simulink library "halin"  (R2021b)
settings: Solver=VariableStepAuto  StartTime=0.0  StopTime=10.0  RelTol=1e-3
undefined symbols (not defined in the file): KHAL_CAN1ABM1E2E_flg, KHAL_CAN1ESC1E2E_flg, KHAL_CAN1ESC5E2E_flg, KHAL_CAN1ESC7E2E_flg, KHAL_CAN1FCM2E2E_flg, KHAL_CAN1FCM3E2E_flg, KHAL_CAN1FCM4E2E_flg, KHAL_CAN3BMS1E2E_flg, KHAL_CAN3BMS6E2E_flg, KHAL_CAN3CCU1E2E_flg, KHAL_CAN3CCU2E2E_flg, KHAL_CAN3MCUF1E2E_flg, KHAL_CAN3MCUR1E2E_flg, KHAL_CAN3Shifter1E2E_flg, TRUE
libraries: simulink x420, FVT_lib x149, hcu_lib x49
(part 3 of 14)

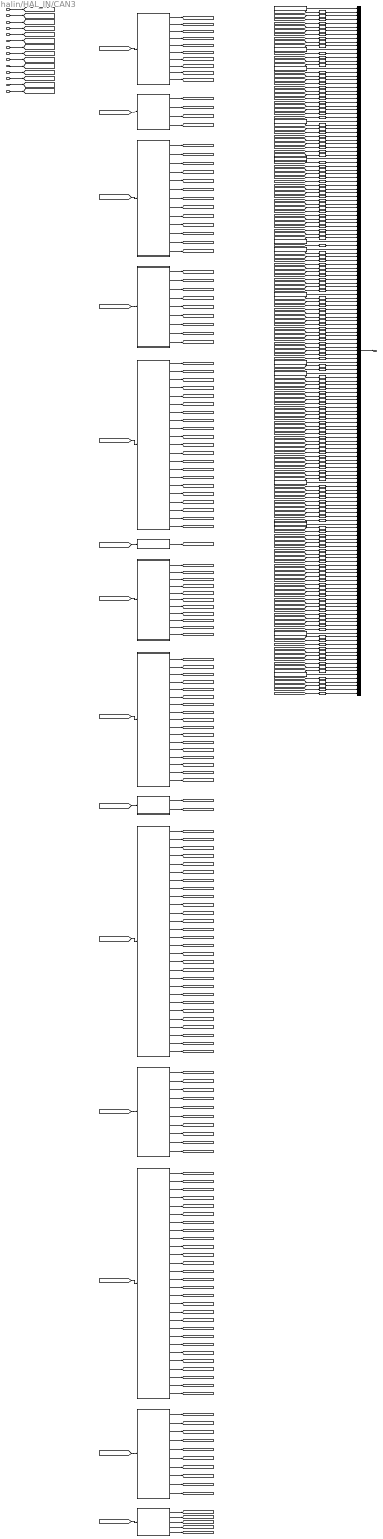
== system halin/HAL_IN/CAN3 ==
  DT_CAN3_SG_BMS1 : Inport
  DT_CAN3_SG_BMS2 : Inport  Port=2
  DT_CAN3_SG_BMS3 : Inport  Port=3
  DT_CAN3_SG_BMS4 : Inport  Port=4
  DT_CAN3_SG_BMS6 : Inport  Port=5
  DT_CAN3_SG_BMS7 : Inport  Port=6
  DT_CAN3_SG_CCU1 : Inport  Port=7
  DT_CAN3_SG_CCU2 : Inport  Port=8
  DT_CAN3_SG_CCU4 : Inport  Port=9
  DT_CAN3_SG_MCU_F1 : Inport  Port=10
  DT_CAN3_SG_MCU_F2 : Inport  Port=11
  DT_CAN3_SG_MCU_R1 : Inport  Port=12
  DT_CAN3_SG_MCU_R2 : Inport  Port=13
  DT_CAN3_SG_Shifter1 : Inport  Port=14
  BMS1 : Subsystem
  BMS2 : Subsystem
  BMS3 : Subsystem
  BMS4 : Subsystem
  BMS6 : Subsystem
  BMS7 : Subsystem
  CCU1 : Subsystem
  CCU2 : Subsystem
  CCU4 : Subsystem
  MCU_F1 : Subsystem
  MCU_F2 : Subsystem
  MCU_R1 : Subsystem
  MCU_R2 : Subsystem
  Shifter1 : Subsystem
  UnitConverter{,1,36..37,40..48,51..52,55,57..59,67,69..70,72,74,78,80..81,88..92,101..102,104..106,126..127,129..131,140..141,143..145,164..165} (49 alike) : DataTypeConversion  OutDataTypeStr=boolean
  UnitConverter{4..31,61..62,64..65,75..77,82,86..87,93,95,98..100,108..114,116..117,122..123,132,134,137..139,147..155,160..161} (70 alike) : DataTypeConversion  OutDataTypeStr=single
  UnitConverter{2..3,32..35,38..39,49..50,53..54,56,60,63,66,68,71,73,79,83..85,94,96..97,103,107,115,118..121,124..125,128,133,135..136,142,146,156..159,162..163,166..168} (50 alike) : DataTypeConversion  OutDataTypeStr=uint8
  VHAL_CANMsgInvalidBMS1_flg : Subsystem  AncestorBlock=FVT_lib/hal/MsgTimeoutJudge_CAN_AUTOSAR
      mask help: MeasumentTrigerEvent
      mask Display: fprintf('MsgTimeoutJudge_CAN\nAUTOSAR');
  VHAL_CANMsgInvalidBMS2_flg : Subsystem  AncestorBlock=FVT_lib/hal/MsgTimeoutJudge_CAN_AUTOSAR
      mask help: MeasumentTrigerEvent
      mask Display: fprintf('MsgTimeoutJudge_CAN\nAUTOSAR');
  VHAL_CANMsgInvalidBMS3_flg : Subsystem  AncestorBlock=FVT_lib/hal/MsgTimeoutJudge_CAN_AUTOSAR
      mask help: MeasumentTrigerEvent
      mask Display: fprintf('MsgTimeoutJudge_CAN\nAUTOSAR');
  VHAL_CANMsgInvalidBMS4_flg : Subsystem  AncestorBlock=FVT_lib/hal/MsgTimeoutJudge_CAN_AUTOSAR
      mask help: MeasumentTrigerEvent
      mask Display: fprintf('MsgTimeoutJudge_CAN\nAUTOSAR');
  VHAL_CANMsgInvalidBMS6_flg : Subsystem  AncestorBlock=FVT_lib/hal/MsgTimeoutJudge_CAN_AUTOSAR
      mask help: MeasumentTrigerEvent
      mask Display: fprintf('MsgTimeoutJudge_CAN\nAUTOSAR');
  VHAL_CANMsgInvalidBMS7_flg : Subsystem  AncestorBlock=FVT_lib/hal/MsgTimeoutJudge_CAN_AUTOSAR
      mask help: MeasumentTrigerEvent
      mask Display: fprintf('MsgTimeoutJudge_CAN\nAUTOSAR');
  VHAL_CANMsgInvalidCCU1_flg : Subsystem  AncestorBlock=FVT_lib/hal/MsgTimeoutJudge_CAN_AUTOSAR
      mask help: MeasumentTrigerEvent
      mask Display: fprintf('MsgTimeoutJudge_CAN\nAUTOSAR');
  VHAL_CANMsgInvalidCCU2_flg : Subsystem  AncestorBlock=FVT_lib/hal/MsgTimeoutJudge_CAN_AUTOSAR
      mask help: MeasumentTrigerEvent
      mask Display: fprintf('MsgTimeoutJudge_CAN\nAUTOSAR');
  VHAL_CANMsgInvalidCCU4_flg : Subsystem  AncestorBlock=FVT_lib/hal/MsgTimeoutJudge_CAN_AUTOSAR
      mask help: MeasumentTrigerEvent
      mask Display: fprintf('MsgTimeoutJudge_CAN\nAUTOSAR');
  VHAL_CANMsgInvalidMCUF1_flg : Subsystem  AncestorBlock=FVT_lib/hal/MsgTimeoutJudge_CAN_AUTOSAR
      mask help: MeasumentTrigerEvent
      mask Display: fprintf('MsgTimeoutJudge_CAN\nAUTOSAR');
  VHAL_CANMsgInvalidMCUF2_flg : Subsystem  AncestorBlock=FVT_lib/hal/MsgTimeoutJudge_CAN_AUTOSAR
      mask help: MeasumentTrigerEvent
      mask Display: fprintf('MsgTimeoutJudge_CAN\nAUTOSAR');
  VHAL_CANMsgInvalidMCUR1_flg : Subsystem  AncestorBlock=FVT_lib/hal/MsgTimeoutJudge_CAN_AUTOSAR
      mask help: MeasumentTrigerEvent
      mask Display: fprintf('MsgTimeoutJudge_CAN\nAUTOSAR');
  VHAL_CANMsgInvalidMCUR2_flg : Subsystem  AncestorBlock=FVT_lib/hal/MsgTimeoutJudge_CAN_AUTOSAR
      mask help: MeasumentTrigerEvent
      mask Display: fprintf('MsgTimeoutJudge_CAN\nAUTOSAR');
  VHAL_CANMsgInvalidShifter1_flg : Subsystem  AncestorBlock=FVT_lib/hal/MsgTimeoutJudge_CAN_AUTOSAR
      mask help: MeasumentTrigerEvent
      mask Display: fprintf('MsgTimeoutJudge_CAN\nAUTOSAR');
  bus_creator : BusCreator  Inputs=183
  HAL_CAN3_outputs : Outport
  wires:
  DT_CAN3_SG_BMS1/1 -> [DT_CAN3_SG_BMS1]
  DT_CAN3_SG_BMS2/1 -> [DT_CAN3_SG_BMS2]
  DT_CAN3_SG_BMS3/1 -> [DT_CAN3_SG_BMS3]
  DT_CAN3_SG_BMS4/1 -> [DT_CAN3_SG_BMS4]
  DT_CAN3_SG_BMS6/1 -> [DT_CAN3_SG_BMS6]
  DT_CAN3_SG_BMS7/1 -> [DT_CAN3_SG_BMS7]
  DT_CAN3_SG_CCU1/1 -> [DT_CAN3_SG_CCU1]
  DT_CAN3_SG_CCU2/1 -> [DT_CAN3_SG_CCU2]
  DT_CAN3_SG_CCU4/1 -> [DT_CAN3_SG_CCU4]
  DT_CAN3_SG_MCU_F1/1 -> [DT_CAN3_SG_MCU_F1]
  DT_CAN3_SG_MCU_F2/1 -> [DT_CAN3_SG_MCU_F2]
  DT_CAN3_SG_MCU_R1/1 -> [DT_CAN3_SG_MCU_R1]
  DT_CAN3_SG_MCU_R2/1 -> [DT_CAN3_SG_MCU_R2]
  DT_CAN3_SG_Shifter1/1 -> [DT_CAN3_SG_Shifter1]
  [DT_CAN3_SG_BMS1] -> BMS1/1(DT_CAN3_SG_BMS1)
  [DT_CAN3_SG_BMS2] -> BMS2/1(DT_CAN3_SG_BMS2)
  [DT_CAN3_SG_BMS3] -> BMS3/1(DT_CAN3_SG_BMS3)
  [DT_CAN3_SG_BMS4] -> BMS4/1(DT_CAN3_SG_BMS4)
  [DT_CAN3_SG_BMS6] -> BMS6/1(DT_CAN3_SG_BMS6)
  [DT_CAN3_SG_BMS7] -> BMS7/1(DT_CAN3_SG_BMS7)
  [DT_CAN3_SG_CCU1] -> CCU1/1(DT_CAN3_SG_CCU1)
  [DT_CAN3_SG_CCU2] -> CCU2/1(DT_CAN3_SG_CCU2)
  [DT_CAN3_SG_CCU4] -> CCU4/1(DT_CAN3_SG_CCU4)
  [DT_CAN3_SG_MCU_F1] -> MCU_F1/1(DT_CAN3_SG_MCU_F1)
  [DT_CAN3_SG_MCU_F2] -> MCU_F2/1(DT_CAN3_SG_MCU_F2)
  [DT_CAN3_SG_MCU_R1] -> MCU_R1/1(DT_CAN3_SG_MCU_R1)
  [DT_CAN3_SG_MCU_R2] -> MCU_R2/1(DT_CAN3_SG_MCU_R2)
  [DT_CAN3_SG_Shifter1] -> Shifter1/1(DT_CAN3_SG_Shifter1)
  bus_creator/1 -> HAL_CAN3_outputs/1
  VHAL_CANMsgInvalidBMS1_flg/1(Out) -> bus_creator/1
  BMS1/1(VHAL_BMS1CSErr_flg) -> [VHAL_BMS1CSErr_flg]
  UnitConverter/1 -> bus_creator/2  "VHAL_BMS1CSErr_flg"
  [VHAL_BMS1CSErr_flg] -> UnitConverter/1
  BMS1/2(VHAL_BMS1RCErr_flg) -> [VHAL_BMS1RCErr_flg]
  UnitConverter1/1 -> bus_creator/3  "VHAL_BMS1RCErr_flg"
  [VHAL_BMS1RCErr_flg] -> UnitConverter1/1
  BMS1/3(VHAL_BMSChckSum1_enum) -> [VHAL_BMSChckSum1_enum]
  UnitConverter2/1 -> bus_creator/4  "VHAL_BMSChckSum1_enum"
  [VHAL_BMSChckSum1_enum] -> UnitConverter2/1
  BMS1/4(VHAL_BMSRolCnct1_enum) -> [VHAL_BMSRolCnct1_enum]
  UnitConverter3/1 -> bus_creator/5  "VHAL_BMSRolCnct1_enum"
  [VHAL_BMSRolCnct1_enum] -> UnitConverter3/1
  BMS1/5(VHAL_HVBPwrAvailChrg_kW) -> [VHAL_HVBPwrAvailChrg_kW]
  UnitConverter4/1 -> bus_creator/6  "VHAL_HVBPwrAvailChrg_kW"
  [VHAL_HVBPwrAvailChrg_kW] -> UnitConverter4/1
  BMS1/6(VHAL_HVBPwrAvailChrg30_kW) -> [VHAL_HVBPwrAvailChrg30_kW]
  UnitConverter5/1 -> bus_creator/7  "VHAL_HVBPwrAvailChrg30_kW"
  [VHAL_HVBPwrAvailChrg30_kW] -> UnitConverter5/1
  BMS1/7(VHAL_HVBPwrAvailChrg60_kW) -> [VHAL_HVBPwrAvailChrg60_kW]
  UnitConverter6/1 -> bus_creator/8  "VHAL_HVBPwrAvailChrg60_kW"
  [VHAL_HVBPwrAvailChrg60_kW] -> UnitConverter6/1
  BMS1/8(VHAL_HVBPwrAvailDchrg_kW) -> [VHAL_HVBPwrAvailDchrg_kW]
  UnitConverter7/1 -> bus_creator/9  "VHAL_HVBPwrAvailDchrg_kW"
  [VHAL_HVBPwrAvailDchrg_kW] -> UnitConverter7/1
  BMS1/9(VHAL_HVBPwrAvailDchrg30_kW) -> [VHAL_HVBPwrAvailDchrg30_kW]
  UnitConverter8/1 -> bus_creator/10  "VHAL_HVBPwrAvailDchrg30_kW"
  [VHAL_HVBPwrAvailDchrg30_kW] -> UnitConverter8/1
  BMS1/10(VHAL_HVBPwrAvailDchrg60_kW) -> [VHAL_HVBPwrAvailDchrg60_kW]
  UnitConverter9/1 -> bus_creator/11  "VHAL_HVBPwrAvailDchrg60_kW"
  [VHAL_HVBPwrAvailDchrg60_kW] -> UnitConverter9/1
  VHAL_CANMsgInvalidBMS2_flg/1(Out) -> bus_creator/12
  BMS2/1(VHAL_HVInVolt_V) -> [VHAL_HVInVolt_V]
  UnitConverter10/1 -> bus_creator/13  "VHAL_HVInVolt_V"
  [VHAL_HVInVolt_V] -> UnitConverter10/1
  BMS2/2(VHAL_LVBattDet12V_V) -> [VHAL_LVBattDet12V_V]
  UnitConverter11/1 -> bus_creator/14  "VHAL_LVBattDet12V_V"
  [VHAL_LVBattDet12V_V] -> UnitConverter11/1
  BMS2/3(VHAL_OBCDCCurLm_A) -> [VHAL_OBCDCCurLm_A]
  UnitConverter12/1 -> bus_creator/15  "VHAL_OBCDCCurLm_A"
  [VHAL_OBCDCCurLm_A] -> UnitConverter12/1
  BMS2/4(VHAL_OBCDCVoltLm_V) -> [VHAL_OBCDCVoltLm_V]
  UnitConverter13/1 -> bus_creator/16  "VHAL_OBCDCVoltLm_V"
  [VHAL_OBCDCVoltLm_V] -> UnitConverter13/1
  VHAL_CANMsgInvalidBMS3_flg/1(Out) -> bus_creator/17
  BMS3/1(VHAL_ACChrgCurrDis_A) -> [VHAL_ACChrgCurrDis_A]
  UnitConverter14/1 -> bus_creator/18  "VHAL_ACChrgCurrDis_A"
  [VHAL_ACChrgCurrDis_A] -> UnitConverter14/1
  BMS3/2(VHAL_HVBChrgPwr_kWh) -> [VHAL_HVBChrgPwr_kWh]
  UnitConverter15/1 -> bus_creator/19  "VHAL_HVBChrgPwr_kWh"
  [VHAL_HVBChrgPwr_kWh] -> UnitConverter15/1
  BMS3/3(VHAL_HVBChrgPwrTotal_kWh) -> [VHAL_HVBChrgPwrTotal_kWh]
  UnitConverter16/1 -> bus_creator/20  "VHAL_HVBChrgPwrTotal_kWh"
  [VHAL_HVBChrgPwrTotal_kWh] -> UnitConverter16/1
  BMS3/4(VHAL_HVBDrvPwr_kWh) -> [VHAL_HVBDrvPwr_kWh]
  UnitConverter17/1 -> bus_creator/21  "VHAL_HVBDrvPwr_kWh"
  [VHAL_HVBDrvPwr_kWh] -> UnitConverter17/1
  BMS3/5(VHAL_HVBDrvPwrTotal_kWh) -> [VHAL_HVBDrvPwrTotal_kWh]
  UnitConverter18/1 -> bus_creator/22  "VHAL_HVBDrvPwrTotal_kWh"
  [VHAL_HVBDrvPwrTotal_kWh] -> UnitConverter18/1
  BMS3/6(VHAL_HVBFullChrgPwr_kWh) -> [VHAL_HVBFullChrgPwr_kWh]
  UnitConverter19/1 -> bus_creator/23  "VHAL_HVBFullChrgPwr_kWh"
  [VHAL_HVBFullChrgPwr_kWh] -> UnitConverter19/1
  BMS3/7(VHAL_HVBIsoImpedenceN_Megaohm) -> [VHAL_HVBIsoImpedenceN_Megaohm]
  UnitConverter20/1 -> bus_creator/24  "VHAL_HVBIsoImpedenceN_Megaohm"
  [VHAL_HVBIsoImpedenceN_Megaohm] -> UnitConverter20/1
  BMS3/8(VHAL_HVBIsoImpedenceP_Megaohm) -> [VHAL_HVBIsoImpedenceP_Megaohm]
  UnitConverter21/1 -> bus_creator/25  "VHAL_HVBIsoImpedenceP_Megaohm"
  [VHAL_HVBIsoImpedenceP_Megaohm] -> UnitConverter21/1
  BMS3/9(VHAL_HVBSOH_pct) -> [VHAL_HVBSOH_pct]
  UnitConverter22/1 -> bus_creator/26  "VHAL_HVBSOH_pct"
  [VHAL_HVBSOH_pct] -> UnitConverter22/1
  BMS3/10(VHAL_HVBattPackVolt_V) -> [VHAL_HVBattPackVolt_V]
  UnitConverter23/1 -> bus_creator/27  "VHAL_HVBattPackVolt_V"
  [VHAL_HVBattPackVolt_V] -> UnitConverter23/1
  BMS3/11(VHAL_HVBattSOC_pct) -> [VHAL_HVBattSOC_pct]
  UnitConverter24/1 -> bus_creator/28  "VHAL_HVBattSOC_pct"
  [VHAL_HVBattSOC_pct] -> UnitConverter24/1
  BMS3/12(VHAL_HVBattSOCDis_pct) -> [VHAL_HVBattSOCDis_pct]
  UnitConverter25/1 -> bus_creator/29  "VHAL_HVBattSOCDis_pct"
  [VHAL_HVBattSOCDis_pct] -> UnitConverter25/1
  BMS3/13(VHAL_RemainChrgTime_min) -> [VHAL_RemainChrgTime_min]
  UnitConverter26/1 -> bus_creator/30  "VHAL_RemainChrgTime_min"
  [VHAL_RemainChrgTime_min] -> UnitConverter26/1
  VHAL_CANMsgInvalidBMS4_flg/1(Out) -> bus_creator/31
  BMS4/1(VHAL_CellTempAvg_C) -> [VHAL_CellTempAvg_C]
  UnitConverter27/1 -> bus_creator/32  "VHAL_CellTempAvg_C"
  [VHAL_CellTempAvg_C] -> UnitConverter27/1
  BMS4/2(VHAL_HVBCellVoltMax_mV) -> [VHAL_HVBCellVoltMax_mV]
  UnitConverter28/1 -> bus_creator/33  "VHAL_HVBCellVoltMax_mV"
  [VHAL_HVBCellVoltMax_mV] -> UnitConverter28/1
  BMS4/3(VHAL_HVBCellVoltMin_mV) -> [VHAL_HVBCellVoltMin_mV]
  UnitConverter29/1 -> bus_creator/34  "VHAL_HVBCellVoltMin_mV"
  [VHAL_HVBCellVoltMin_mV] -> UnitConverter29/1
  BMS4/4(VHAL_HVBMTempMax_C) -> [VHAL_HVBMTempMax_C]
  UnitConverter30/1 -> bus_creator/35  "VHAL_HVBMTempMax_C"
  [VHAL_HVBMTempMax_C] -> UnitConverter30/1
  BMS4/5(VHAL_HVBMTempMin_C) -> [VHAL_HVBMTempMin_C]
  UnitConverter31/1 -> bus_creator/36  "VHAL_HVBMTempMin_C"
  [VHAL_HVBMTempMin_C] -> UnitConverter31/1
  BMS4/6(VHAL_MaxCellTempNum_enum) -> [VHAL_MaxCellTempNum_enum]
  UnitConverter32/1 -> bus_creator/37  "VHAL_MaxCellTempNum_enum"
  [VHAL_MaxCellTempNum_enum] -> UnitConverter32/1
  BMS4/7(VHAL_MaxCellVoltNum_enum) -> [VHAL_MaxCellVoltNum_enum]
  UnitConverter33/1 -> bus_creator/38  "VHAL_MaxCellVoltNum_enum"
  [VHAL_MaxCellVoltNum_enum] -> UnitConverter33/1
  BMS4/8(VHAL_MinCellTempNum_enum) -> [VHAL_MinCellTempNum_enum]
  UnitConverter34/1 -> bus_creator/39  "VHAL_MinCellTempNum_enum"
  [VHAL_MinCellTempNum_enum] -> UnitConverter34/1
  BMS4/9(VHAL_MinCellVoltNum_enum) -> [VHAL_MinCellVoltNum_enum]
  UnitConverter35/1 -> bus_creator/40  "VHAL_MinCellVoltNum_enum"
  [VHAL_MinCellVoltNum_enum] -> UnitConverter35/1
  VHAL_CANMsgInvalidBMS6_flg/1(Out) -> bus_creator/41
  BMS6/1(VHAL_BMS6CSErr_flg) -> [VHAL_BMS6CSErr_flg]
  UnitConverter36/1 -> bus_creator/42  "VHAL_BMS6CSErr_flg"
  [VHAL_BMS6CSErr_flg] -> UnitConverter36/1
  BMS6/2(VHAL_BMS6RCErr_flg) -> [VHAL_BMS6RCErr_flg]
  UnitConverter37/1 -> bus_creator/43  "VHAL_BMS6RCErr_flg"
  [VHAL_BMS6RCErr_flg] -> UnitConverter37/1
  BMS6/3(VHAL_BMSChckSum_enum) -> [VHAL_BMSChckSum_enum]
  UnitConverter38/1 -> bus_creator/44  "VHAL_BMSChckSum_enum"
  [VHAL_BMSChckSum_enum] -> UnitConverter38/1
  BMS6/4(VHAL_BMSRolCnct_enum) -> [VHAL_BMSRolCnct_enum]
  UnitConverter39/1 -> bus_creator/45  "VHAL_BMSRolCnct_enum"
  [VHAL_BMSRolCnct_enum] -> UnitConverter39/1
  BMS6/5(VHAL_BMSREADY_flg) -> [VHAL_BMSREADY_flg]
  UnitConverter40/1 -> bus_creator/46  "VHAL_BMSREADY_flg"
  [VHAL_BMSREADY_flg] -> UnitConverter40/1
  BMS6/6(VHAL_BMSWarn1_flg) -> [VHAL_BMSWarn1_flg]
  UnitConverter41/1 -> bus_creator/47  "VHAL_BMSWarn1_flg"
  [VHAL_BMSWarn1_flg] -> UnitConverter41/1
  BMS6/7(VHAL_BMSWarn2_flg) -> [VHAL_BMSWarn2_flg]
  UnitConverter42/1 -> bus_creator/48  "VHAL_BMSWarn2_flg"
  [VHAL_BMSWarn2_flg] -> UnitConverter42/1
  BMS6/8(VHAL_BMSWarn3_flg) -> [VHAL_BMSWarn3_flg]
  UnitConverter43/1 -> bus_creator/49  "VHAL_BMSWarn3_flg"
  [VHAL_BMSWarn3_flg] -> UnitConverter43/1
  BMS6/9(VHAL_BMSWarn4_flg) -> [VHAL_BMSWarn4_flg]
  UnitConverter44/1 -> bus_creator/50  "VHAL_BMSWarn4_flg"
  [VHAL_BMSWarn4_flg] -> UnitConverter44/1
  BMS6/10(VHAL_BMSWarn5_flg) -> [VHAL_BMSWarn5_flg]
  UnitConverter45/1 -> bus_creator/51  "VHAL_BMSWarn5_flg"
  [VHAL_BMSWarn5_flg] -> UnitConverter45/1
  BMS6/11(VHAL_BMSWarn6_flg) -> [VHAL_BMSWarn6_flg]
  UnitConverter46/1 -> bus_creator/52  "VHAL_BMSWarn6_flg"
  [VHAL_BMSWarn6_flg] -> UnitConverter46/1
  BMS6/12(VHAL_BMSWarn7_flg) -> [VHAL_BMSWarn7_flg]
  UnitConverter47/1 -> bus_creator/53  "VHAL_BMSWarn7_flg"
  [VHAL_BMSWarn7_flg] -> UnitConverter47/1
  BMS6/13(VHAL_BMSWarn8_flg) -> [VHAL_BMSWarn8_flg]
  UnitConverter48/1 -> bus_creator/54  "VHAL_BMSWarn8_flg"
  [VHAL_BMSWarn8_flg] -> UnitConverter48/1
  BMS6/14(VHAL_ChrgPlugSta_enum) -> [VHAL_ChrgPlugSta_enum]
  UnitConverter49/1 -> bus_creator/55  "VHAL_ChrgPlugSta_enum"
  [VHAL_ChrgPlugSta_enum] -> UnitConverter49/1
  BMS6/15(VHAL_ExtChrgSta_enum) -> [VHAL_ExtChrgSta_enum]
  UnitConverter50/1 -> bus_creator/56  "VHAL_ExtChrgSta_enum"
  [VHAL_ExtChrgSta_enum] -> UnitConverter50/1
  BMS6/16(VHAL_HVBContactorSta_flg) -> [VHAL_HVBContactorSta_flg]
  UnitConverter51/1 -> bus_creator/57  "VHAL_HVBContactorSta_flg"
  [VHAL_HVBContactorSta_flg] -> UnitConverter51/1
  BMS6/17(VHAL_HVBHVILErr_flg) -> [VHAL_HVBHVILErr_flg]
  UnitConverter52/1 -> bus_creator/58  "VHAL_HVBHVILErr_flg"
  [VHAL_HVBHVILErr_flg] -> UnitConverter52/1
  BMS6/18(VHAL_HVBPreheatPrecoolSta_enum) -> [VHAL_HVBPreheatPrecoolSta_enum]
  UnitConverter53/1 -> bus_creator/59  "VHAL_HVBPreheatPrecoolSta_enum"
  [VHAL_HVBPreheatPrecoolSta_enum] -> UnitConverter53/1
  BMS6/19(VHAL_HVBattReady4Pre_enum) -> [VHAL_HVBattReady4Pre_enum]
  UnitConverter54/1 -> bus_creator/60  "VHAL_HVBattReady4Pre_enum"
  [VHAL_HVBattReady4Pre_enum] -> UnitConverter54/1
  BMS6/20(VHAL_HVILSta_flg) -> [VHAL_HVILSta_flg]
  UnitConverter55/1 -> bus_creator/61  "VHAL_HVILSta_flg"
  [VHAL_HVILSta_flg] -> UnitConverter55/1
  BMS6/21(VHAL_V2LSta_enum) -> [VHAL_V2LSta_enum]
  UnitConverter56/1 -> bus_creator/62  "VHAL_V2LSta_enum"
  [VHAL_V2LSta_enum] -> UnitConverter56/1
  VHAL_CANMsgInvalidBMS7_flg/1(Out) -> bus_creator/63
  BMS7/1(VHAL_HVBattErr_flg) -> [VHAL_HVBattErr_flg]
  UnitConverter57/1 -> bus_creator/64  "VHAL_HVBattErr_flg"
  [VHAL_HVBattErr_flg] -> UnitConverter57/1
  VHAL_CANMsgInvalidCCU1_flg/1(Out) -> bus_creator/65
  CCU1/1(VHAL_CCU1CSErr_flg) -> [VHAL_CCU1CSErr_flg]
  UnitConverter58/1 -> bus_creator/66  "VHAL_CCU1CSErr_flg"
  [VHAL_CCU1CSErr_flg] -> UnitConverter58/1
  CCU1/2(VHAL_CCU1RCErr_flg) -> [VHAL_CCU1RCErr_flg]
  UnitConverter59/1 -> bus_creator/67  "VHAL_CCU1RCErr_flg"
  [VHAL_CCU1RCErr_flg] -> UnitConverter59/1
  CCU1/3(VHAL_CSCCU1_enum) -> [VHAL_CSCCU1_enum]
  UnitConverter60/1 -> bus_creator/68  "VHAL_CSCCU1_enum"
  [VHAL_CSCCU1_enum] -> UnitConverter60/1
  CCU1/4(VHAL_DCDCAuxVolt_V) -> [VHAL_DCDCAuxVolt_V]
  UnitConverter61/1 -> bus_creator/69  "VHAL_DCDCAuxVolt_V"
  [VHAL_DCDCAuxVolt_V] -> UnitConverter61/1
  CCU1/5(VHAL_DCDCInVoltInf_V) -> [VHAL_DCDCInVoltInf_V]
  UnitConverter62/1 -> bus_creator/70  "VHAL_DCDCInVoltInf_V"
  [VHAL_DCDCInVoltInf_V] -> UnitConverter62/1
  CCU1/6(VHAL_DCDCPreCompleted_enum) -> [VHAL_DCDCPreCompleted_enum]
  UnitConverter63/1 -> bus_creator/71  "VHAL_DCDCPreCompleted_enum"
  [VHAL_DCDCPreCompleted_enum] -> UnitConverter63/1
  CCU1/7(VHAL_OBCDCCurrInf_A) -> [VHAL_OBCDCCurrInf_A]
  UnitConverter64/1 -> bus_creator/72  "VHAL_OBCDCCurrInf_A"
  [VHAL_OBCDCCurrInf_A] -> UnitConverter64/1
  CCU1/8(VHAL_OBCDCVoltInf_V) -> [VHAL_OBCDCVoltInf_V]
  UnitConverter65/1 -> bus_creator/73  "VHAL_OBCDCVoltInf_V"
  [VHAL_OBCDCVoltInf_V] -> UnitConverter65/1
  CCU1/9(VHAL_OBCPreCompleted_enum) -> [VHAL_OBCPreCompleted_enum]
  UnitConverter66/1 -> bus_creator/74  "VHAL_OBCPreCompleted_enum"
  [VHAL_OBCPreCompleted_enum] -> UnitConverter66/1
  CCU1/10(VHAL_OBCWakeup4Plugin_flg) -> [VHAL_OBCWakeup4Plugin_flg]
  UnitConverter67/1 -> bus_creator/75  "VHAL_OBCWakeup4Plugin_flg"
  [VHAL_OBCWakeup4Plugin_flg] -> UnitConverter67/1
  CCU1/11(VHAL_RCCCU1_enum) -> [VHAL_RCCCU1_enum]
  UnitConverter68/1 -> bus_creator/76  "VHAL_RCCCU1_enum"
  [VHAL_RCCCU1_enum] -> UnitConverter68/1
  VHAL_CANMsgInvalidCCU2_flg/1(Out) -> bus_creator/77
  CCU2/1(VHAL_CCU2CSErr_flg) -> [VHAL_CCU2CSErr_flg]
  UnitConverter69/1 -> bus_creator/78  "VHAL_CCU2CSErr_flg"
  [VHAL_CCU2CSErr_flg] -> UnitConverter69/1
  CCU2/2(VHAL_CCU2RCErr_flg) -> [VHAL_CCU2RCErr_flg]
  UnitConverter70/1 -> bus_creator/79  "VHAL_CCU2RCErr_flg"
  [VHAL_CCU2RCErr_flg] -> UnitConverter70/1
  CCU2/3(VHAL_CSCCU2_enum) -> [VHAL_CSCCU2_enum]
  UnitConverter71/1 -> bus_creator/80  "VHAL_CSCCU2_enum"
  [VHAL_CSCCU2_enum] -> UnitConverter71/1
  CCU2/4(VHAL_DCDCEnaSta_flg) -> [VHAL_DCDCEnaSta_flg]
  UnitConverter72/1 -> bus_creator/81  "VHAL_DCDCEnaSta_flg"
  [VHAL_DCDCEnaSta_flg] -> UnitConverter72/1
  CCU2/5(VHAL_DCDCFaultSta_enum) -> [VHAL_DCDCFaultSta_enum]
  UnitConverter73/1 -> bus_creator/82  "VHAL_DCDCFaultSta_enum"
  [VHAL_DCDCFaultSta_enum] -> UnitConverter73/1
  CCU2/6(VHAL_DCDCReady4Pre_flg) -> [VHAL_DCDCReady4Pre_flg]
  UnitConverter74/1 -> bus_creator/83  "VHAL_DCDCReady4Pre_flg"
  [VHAL_DCDCReady4Pre_flg] -> UnitConverter74/1
  CCU2/7(VHAL_DCDCTemp_C) -> [VHAL_DCDCTemp_C]
  UnitConverter75/1 -> bus_creator/84  "VHAL_DCDCTemp_C"
  [VHAL_DCDCTemp_C] -> UnitConverter75/1
  CCU2/8(VHAL_OBCACCurrInf_A) -> [VHAL_OBCACCurrInf_A]
  UnitConverter76/1 -> bus_creator/85  "VHAL_OBCACCurrInf_A"
  [VHAL_OBCACCurrInf_A] -> UnitConverter76/1
  CCU2/9(VHAL_OBCACVoltInf_V) -> [VHAL_OBCACVoltInf_V]
  UnitConverter77/1 -> bus_creator/86  "VHAL_OBCACVoltInf_V"
  [VHAL_OBCACVoltInf_V] -> UnitConverter77/1
  CCU2/10(VHAL_OBCEnaSta_flg) -> [VHAL_OBCEnaSta_flg]
  UnitConverter78/1 -> bus_creator/87  "VHAL_OBCEnaSta_flg"
  [VHAL_OBCEnaSta_flg] -> UnitConverter78/1
  CCU2/11(VHAL_OBCFaultSta_enum) -> [VHAL_OBCFaultSta_enum]
  UnitConverter79/1 -> bus_creator/88  "VHAL_OBCFaultSta_enum"
  [VHAL_OBCFaultSta_enum] -> UnitConverter79/1
  CCU2/12(VHAL_OBCPluginSta_flg) -> [VHAL_OBCPluginSta_flg]
  UnitConverter80/1 -> bus_creator/89  "VHAL_OBCPluginSta_flg"
  [VHAL_OBCPluginSta_flg] -> UnitConverter80/1
  CCU2/13(VHAL_OBCReady4Pre_flg) -> [VHAL_OBCReady4Pre_flg]
  UnitConverter81/1 -> bus_creator/90  "VHAL_OBCReady4Pre_flg"
  [VHAL_OBCReady4Pre_flg] -> UnitConverter81/1
  CCU2/14(VHAL_OBCTemp_C) -> [VHAL_OBCTemp_C]
  UnitConverter82/1 -> bus_creator/91  "VHAL_OBCTemp_C"
  [VHAL_OBCTemp_C] -> UnitConverter82/1
  CCU2/15(VHAL_OBCV2LSta_enum) -> [VHAL_OBCV2LSta_enum]
  UnitConverter83/1 -> bus_creator/92  "VHAL_OBCV2LSta_enum"
  [VHAL_OBCV2LSta_enum] -> UnitConverter83/1
  CCU2/16(VHAL_OBCACCurLim_enum) -> [VHAL_OBCACCurLim_enum]
  UnitConverter84/1 -> bus_creator/93  "VHAL_OBCACCurLim_enum"
  [VHAL_OBCACCurLim_enum] -> UnitConverter84/1
  CCU2/17(VHAL_RCCCU2_enum) -> [VHAL_RCCCU2_enum]
  UnitConverter85/1 -> bus_creator/94  "VHAL_RCCCU2_enum"
  [VHAL_RCCCU2_enum] -> UnitConverter85/1
  VHAL_CANMsgInvalidCCU4_flg/1(Out) -> bus_creator/95
  CCU4/1(VHAL_DCDCAuxCur_A) -> [VHAL_DCDCAuxCur_A]
  UnitConverter86/1 -> bus_creator/96  "VHAL_DCDCAuxCur_A"
  [VHAL_DCDCAuxCur_A] -> UnitConverter86/1
  CCU4/2(VHAL_DCDCHVCur_A) -> [VHAL_DCDCHVCur_A]
  UnitConverter87/1 -> bus_creator/97  "VHAL_DCDCHVCur_A"
  [VHAL_DCDCHVCur_A] -> UnitConverter87/1
  VHAL_CANMsgInvalidMCUF1_flg/1(Out) -> bus_creator/98
  MCU_F1/1(VHAL_MCUF1CSErr_flg) -> [VHAL_MCUF1CSErr_flg]
  UnitConverter88/1 -> bus_creator/99  "VHAL_MCUF1CSErr_flg"
  [VHAL_MCUF1CSErr_flg] -> UnitConverter88/1
  MCU_F1/2(VHAL_MCUF1RCErr_flg) -> [VHAL_MCUF1RCErr_flg]
  UnitConverter89/1 -> bus_creator/100  "VHAL_MCUF1RCErr_flg"
  [VHAL_MCUF1RCErr_flg] -> UnitConverter89/1
  MCU_F1/3(VHAL_FrActvDmpDisabSta_flg) -> [VHAL_FrActvDmpDisabSta_flg]
  UnitConverter90/1 -> bus_creator/101  "VHAL_FrActvDmpDisabSta_flg"
  [VHAL_FrActvDmpDisabSta_flg] -> UnitConverter90/1
  MCU_F1/4(VHAL_FrEDUDrtSta_flg) -> [VHAL_FrEDUDrtSta_flg]
  UnitConverter91/1 -> bus_creator/102  "VHAL_FrEDUDrtSta_flg"
  [VHAL_FrEDUDrtSta_flg] -> UnitConverter91/1
  MCU_F1/5(VHAL_FrEDUOpratingSta_flg) -> [VHAL_FrEDUOpratingSta_flg]
  UnitConverter92/1 -> bus_creator/103  "VHAL_FrEDUOpratingSta_flg"
  [VHAL_FrEDUOpratingSta_flg] -> UnitConverter92/1
  MCU_F1/6(VHAL_FrEDURealTMTq_Nm) -> [VHAL_FrEDURealTMTq_Nm]
  UnitConverter93/1 -> bus_creator/104  "VHAL_FrEDURealTMTq_Nm"
  [VHAL_FrEDURealTMTq_Nm] -> UnitConverter93/1
  MCU_F1/7(VHAL_FrEDURotateDirction_enum) -> [VHAL_FrEDURotateDirction_enum]
  UnitConverter94/1 -> bus_creator/105  "VHAL_FrEDURotateDirction_enum"
  [VHAL_FrEDURotateDirction_enum] -> UnitConverter94/1
  MCU_F1/8(VHAL_FrEDUTqReqFbk_Nm) -> [VHAL_FrEDUTqReqFbk_Nm]
  UnitConverter95/1 -> bus_creator/106  "VHAL_FrEDUTqReqFbk_Nm"
  [VHAL_FrEDUTqReqFbk_Nm] -> UnitConverter95/1
  MCU_F1/9(VHAL_FrMCU1Chksum_enum) -> [VHAL_FrMCU1Chksum_enum]
  UnitConverter96/1 -> bus_creator/107  "VHAL_FrMCU1Chksum_enum"
  [VHAL_FrMCU1Chksum_enum] -> UnitConverter96/1
  MCU_F1/10(VHAL_FrMCU1RolCnt_enum) -> [VHAL_FrMCU1RolCnt_enum]
  UnitConverter97/1 -> bus_creator/108  "VHAL_FrMCU1RolCnt_enum"
  [VHAL_FrMCU1RolCnt_enum] -> UnitConverter97/1
  MCU_F1/11(VHAL_FrMCUBAT_V) -> [VHAL_FrMCUBAT_V]
  UnitConverter98/1 -> bus_creator/109  "VHAL_FrMCUBAT_V"
  [VHAL_FrMCUBAT_V] -> UnitConverter98/1
  MCU_F1/12(VHAL_FrMCUDCBusCurr_A) -> [VHAL_FrMCUDCBusCurr_A]
  UnitConverter99/1 -> bus_creator/110  "VHAL_FrMCUDCBusCurr_A"
  [VHAL_FrMCUDCBusCurr_A] -> UnitConverter99/1
  MCU_F1/13(VHAL_FrMCUDCBusVolt_V) -> [VHAL_FrMCUDCBusVolt_V]
  UnitConverter100/1 -> bus_creator/111  "VHAL_FrMCUDCBusVolt_V"
  [VHAL_FrMCUDCBusVolt_V] -> UnitConverter100/1
  MCU_F1/14(VHAL_FrMCUDischrgSta_flg) -> [VHAL_FrMCUDischrgSta_flg]
  UnitConverter101/1 -> bus_creator/112  "VHAL_FrMCUDischrgSta_flg"
  [VHAL_FrMCUDischrgSta_flg] -> UnitConverter101/1
  MCU_F1/15(VHAL_FrMCUEnaSta_flg) -> [VHAL_FrMCUEnaSta_flg]
  UnitConverter102/1 -> bus_creator/113  "VHAL_FrMCUEnaSta_flg"
  [VHAL_FrMCUEnaSta_flg] -> UnitConverter102/1
  MCU_F1/16(VHAL_FrMCUErr_enum) -> [VHAL_FrMCUErr_enum]
  UnitConverter103/1 -> bus_creator/114  "VHAL_FrMCUErr_enum"
  [VHAL_FrMCUErr_enum] -> UnitConverter103/1
  MCU_F1/17(VHAL_FrMCUIGNsta_flg) -> [VHAL_FrMCUIGNsta_flg]
  UnitConverter104/1 -> bus_creator/115  "VHAL_FrMCUIGNsta_flg"
  [VHAL_FrMCUIGNsta_flg] -> UnitConverter104/1
  MCU_F1/18(VHAL_FrMCUReady_flg) -> [VHAL_FrMCUReady_flg]
  UnitConverter105/1 -> bus_creator/116  "VHAL_FrMCUReady_flg"
  [VHAL_FrMCUReady_flg] -> UnitConverter105/1
  MCU_F1/19(VHAL_FrMCUReady4Pre_flg) -> [VHAL_FrMCUReady4Pre_flg]
  UnitConverter106/1 -> bus_creator/117  "VHAL_FrMCUReady4Pre_flg"
  [VHAL_FrMCUReady4Pre_flg] -> UnitConverter106/1
  MCU_F1/20(VHAL_FrMCUSysSta_enum) -> [VHAL_FrMCUSysSta_enum]
  UnitConverter107/1 -> bus_creator/118  "VHAL_FrMCUSysSta_enum"
  [VHAL_FrMCUSysSta_enum] -> UnitConverter107/1
  MCU_F1/21(VHAL_FrMCUTemp_C) -> [VHAL_FrMCUTemp_C]
  UnitConverter108/1 -> bus_creator/119  "VHAL_FrMCUTemp_C"
  [VHAL_FrMCUTemp_C] -> UnitConverter108/1
  MCU_F1/22(VHAL_FrMotorAvailTq_Nm) -> [VHAL_FrMotorAvailTq_Nm]
  UnitConverter109/1 -> bus_creator/120  "VHAL_FrMotorAvailTq_Nm"
  [VHAL_FrMotorAvailTq_Nm] -> UnitConverter109/1
  MCU_F1/23(VHAL_FrRegenAvailTq_Nm) -> [VHAL_FrRegenAvailTq_Nm]
  UnitConverter110/1 -> bus_creator/121  "VHAL_FrRegenAvailTq_Nm"
  [VHAL_FrRegenAvailTq_Nm] -> UnitConverter110/1
  MCU_F1/24(VHAL_FrTMSpd_rpm) -> [VHAL_FrTMSpd_rpm]
  UnitConverter111/1 -> bus_creator/122  "VHAL_FrTMSpd_rpm"
  [VHAL_FrTMSpd_rpm] -> UnitConverter111/1
  MCU_F1/25(VHAL_FrTMTemp_C) -> [VHAL_FrTMTemp_C]
  UnitConverter112/1 -> bus_creator/123  "VHAL_FrTMTemp_C"
  [VHAL_FrTMTemp_C] -> UnitConverter112/1
  MCU_F1/26(VHAL_FrTMid_A) -> [VHAL_FrTMid_A]
  UnitConverter113/1 -> bus_creator/124  "VHAL_FrTMid_A"
  [VHAL_FrTMid_A] -> UnitConverter113/1
  MCU_F1/27(VHAL_FrTMiq_A) -> [VHAL_FrTMiq_A]
  UnitConverter114/1 -> bus_creator/125  "VHAL_FrTMiq_A"
  [VHAL_FrTMiq_A] -> UnitConverter114/1
  MCU_F1/28(VHAL_MCUWarnF_enum) -> [VHAL_MCUWarnF_enum]
  UnitConverter115/1 -> bus_creator/126  "VHAL_MCUWarnF_enum"
  [VHAL_MCUWarnF_enum] -> UnitConverter115/1
  VHAL_CANMsgInvalidMCUF2_flg/1(Out) -> bus_creator/127
  MCU_F2/1(VHAL_FrCoolanttempReq_C) -> [VHAL_FrCoolanttempReq_C]
  UnitConverter116/1 -> bus_creator/128  "VHAL_FrCoolanttempReq_C"
  [VHAL_FrCoolanttempReq_C] -> UnitConverter116/1
  MCU_F2/2(VHAL_FrEOPSpdSet_rpm) -> [VHAL_FrEOPSpdSet_rpm]
  UnitConverter117/1 -> bus_creator/129  "VHAL_FrEOPSpdSet_rpm"
  [VHAL_FrEOPSpdSet_rpm] -> UnitConverter117/1
  MCU_F2/3(VHAL_FrFailcode1_enum) -> [VHAL_FrFailcode1_enum]
  UnitConverter118/1 -> bus_creator/130  "VHAL_FrFailcode1_enum"
  [VHAL_FrFailcode1_enum] -> UnitConverter118/1
  MCU_F2/4(VHAL_FrFailcode2_enum) -> [VHAL_FrFailcode2_enum]
  UnitConverter119/1 -> bus_creator/131  "VHAL_FrFailcode2_enum"
  [VHAL_FrFailcode2_enum] -> UnitConverter119/1
  MCU_F2/5(VHAL_FrFailcodehistory1_enum) -> [VHAL_FrFailcodehistory1_enum]
  UnitConverter120/1 -> bus_creator/132  "VHAL_FrFailcodehistory1_enum"
  [VHAL_FrFailcodehistory1_enum] -> UnitConverter120/1
  MCU_F2/6(VHAL_FrFailcodehistory2_enum) -> [VHAL_FrFailcodehistory2_enum]
  UnitConverter121/1 -> bus_creator/133  "VHAL_FrFailcodehistory2_enum"
  [VHAL_FrFailcodehistory2_enum] -> UnitConverter121/1
  MCU_F2/7(VHAL_FrLLCTemp_C) -> [VHAL_FrLLCTemp_C]
  UnitConverter122/1 -> bus_creator/134  "VHAL_FrLLCTemp_C"
  [VHAL_FrLLCTemp_C] -> UnitConverter122/1
  MCU_F2/8(VHAL_FrLLCflowReq_Lpmin) -> [VHAL_FrLLCflowReq_Lpmin]
  UnitConverter123/1 -> bus_creator/135  "VHAL_FrLLCflowReq_Lpmin"
  [VHAL_FrLLCflowReq_Lpmin] -> UnitConverter123/1
  MCU_F2/9(VHAL_FrMCUTempWarn_enum) -> [VHAL_FrMCUTempWarn_enum]
  UnitConverter124/1 -> bus_creator/136  "VHAL_FrMCUTempWarn_enum"
  [VHAL_FrMCUTempWarn_enum] -> UnitConverter124/1
  MCU_F2/10(VHAL_FrTMTempWarn_enum) -> [VHAL_FrTMTempWarn_enum]
  UnitConverter125/1 -> bus_creator/137  "VHAL_FrTMTempWarn_enum"
  [VHAL_FrTMTempWarn_enum] -> UnitConverter125/1
  VHAL_CANMsgInvalidMCUR1_flg/1(Out) -> bus_creator/138
  MCU_R1/1(VHAL_MCUR1CSErr_flg) -> [VHAL_MCUR1CSErr_flg]
  UnitConverter126/1 -> bus_creator/139  "VHAL_MCUR1CSErr_flg"
  [VHAL_MCUR1CSErr_flg] -> UnitConverter126/1
  MCU_R1/2(VHAL_MCUR1RCErr_flg) -> [VHAL_MCUR1RCErr_flg]
  UnitConverter127/1 -> bus_creator/140  "VHAL_MCUR1RCErr_flg"
  [VHAL_MCUR1RCErr_flg] -> UnitConverter127/1
  MCU_R1/3(VHAL_MCUWarnR_enum) -> [VHAL_MCUWarnR_enum]
  UnitConverter128/1 -> bus_creator/141  "VHAL_MCUWarnR_enum"
  [VHAL_MCUWarnR_enum] -> UnitConverter128/1
  MCU_R1/4(VHAL_RrActvDmpDisabSta_flg) -> [VHAL_RrActvDmpDisabSta_flg]
  UnitConverter129/1 -> bus_creator/142  "VHAL_RrActvDmpDisabSta_flg"
  [VHAL_RrActvDmpDisabSta_flg] -> UnitConverter129/1
  MCU_R1/5(VHAL_RrEDUDrtSta_flg) -> [VHAL_RrEDUDrtSta_flg]
  UnitConverter130/1 -> bus_creator/143  "VHAL_RrEDUDrtSta_flg"
  [VHAL_RrEDUDrtSta_flg] -> UnitConverter130/1
  MCU_R1/6(VHAL_RrEDUOpratingSta_flg) -> [VHAL_RrEDUOpratingSta_flg]
  UnitConverter131/1 -> bus_creator/144  "VHAL_RrEDUOpratingSta_flg"
  [VHAL_RrEDUOpratingSta_flg] -> UnitConverter131/1
  MCU_R1/7(VHAL_RrEDURealTMTq_Nm) -> [VHAL_RrEDURealTMTq_Nm]
  UnitConverter132/1 -> bus_creator/145  "VHAL_RrEDURealTMTq_Nm"
  [VHAL_RrEDURealTMTq_Nm] -> UnitConverter132/1
  MCU_R1/8(VHAL_RrEDURotateDirction_enum) -> [VHAL_RrEDURotateDirction_enum]
  UnitConverter133/1 -> bus_creator/146  "VHAL_RrEDURotateDirction_enum"
  [VHAL_RrEDURotateDirction_enum] -> UnitConverter133/1
  MCU_R1/9(VHAL_RrEDUTqReqFbk_Nm) -> [VHAL_RrEDUTqReqFbk_Nm]
  UnitConverter134/1 -> bus_creator/147  "VHAL_RrEDUTqReqFbk_Nm"
  [VHAL_RrEDUTqReqFbk_Nm] -> UnitConverter134/1
  MCU_R1/10(VHAL_RrMCU1Chksum_enum) -> [VHAL_RrMCU1Chksum_enum]
  UnitConverter135/1 -> bus_creator/148  "VHAL_RrMCU1Chksum_enum"
  [VHAL_RrMCU1Chksum_enum] -> UnitConverter135/1
  MCU_R1/11(VHAL_RrMCU1RolCnt_enum) -> [VHAL_RrMCU1RolCnt_enum]
  UnitConverter136/1 -> bus_creator/149  "VHAL_RrMCU1RolCnt_enum"
  [VHAL_RrMCU1RolCnt_enum] -> UnitConverter136/1
  MCU_R1/12(VHAL_RrMCUBAT_V) -> [VHAL_RrMCUBAT_V]
  UnitConverter137/1 -> bus_creator/150  "VHAL_RrMCUBAT_V"
  [VHAL_RrMCUBAT_V] -> UnitConverter137/1
  MCU_R1/13(VHAL_RrMCUDCBusCurr_A) -> [VHAL_RrMCUDCBusCurr_A]
  UnitConverter138/1 -> bus_creator/151  "VHAL_RrMCUDCBusCurr_A"
  [VHAL_RrMCUDCBusCurr_A] -> UnitConverter138/1
  MCU_R1/14(VHAL_RrMCUDCBusVolt_V) -> [VHAL_RrMCUDCBusVolt_V]
  UnitConverter139/1 -> bus_creator/152  "VHAL_RrMCUDCBusVolt_V"
  [VHAL_RrMCUDCBusVolt_V] -> UnitConverter139/1
  MCU_R1/15(VHAL_RrMCUDischrgSta_flg) -> [VHAL_RrMCUDischrgSta_flg]
  UnitConverter140/1 -> bus_creator/153  "VHAL_RrMCUDischrgSta_flg"
  [VHAL_RrMCUDischrgSta_flg] -> UnitConverter140/1
  MCU_R1/16(VHAL_RrMCUEnaSta_flg) -> [VHAL_RrMCUEnaSta_flg]
  UnitConverter141/1 -> bus_creator/154  "VHAL_RrMCUEnaSta_flg"
  [VHAL_RrMCUEnaSta_flg] -> UnitConverter141/1
  MCU_R1/17(VHAL_RrMCUErr_enum) -> [VHAL_RrMCUErr_enum]
  UnitConverter142/1 -> bus_creator/155  "VHAL_RrMCUErr_enum"
  [VHAL_RrMCUErr_enum] -> UnitConverter142/1
  MCU_R1/18(VHAL_RrMCUIGNsta_flg) -> [VHAL_RrMCUIGNsta_flg]
  UnitConverter143/1 -> bus_creator/156  "VHAL_RrMCUIGNsta_flg"
  [VHAL_RrMCUIGNsta_flg] -> UnitConverter143/1
  MCU_R1/19(VHAL_RrMCUReady_flg) -> [VHAL_RrMCUReady_flg]
  UnitConverter144/1 -> bus_creator/157  "VHAL_RrMCUReady_flg"
  [VHAL_RrMCUReady_flg] -> UnitConverter144/1
  MCU_R1/20(VHAL_RrMCUReady4Pre_flg) -> [VHAL_RrMCUReady4Pre_flg]
  UnitConverter145/1 -> bus_creator/158  "VHAL_RrMCUReady4Pre_flg"
  [VHAL_RrMCUReady4Pre_flg] -> UnitConverter145/1
  MCU_R1/21(VHAL_RrMCUSysSta_enum) -> [VHAL_RrMCUSysSta_enum]
  UnitConverter146/1 -> bus_creator/159  "VHAL_RrMCUSysSta_enum"
  [VHAL_RrMCUSysSta_enum] -> UnitConverter146/1
  MCU_R1/22(VHAL_RrMCUTemp_C) -> [VHAL_RrMCUTemp_C]
  UnitConverter147/1 -> bus_creator/160  "VHAL_RrMCUTemp_C"
  [VHAL_RrMCUTemp_C] -> UnitConverter147/1
  MCU_R1/23(VHAL_RrMotorAvailTq_Nm) -> [VHAL_RrMotorAvailTq_Nm]
  UnitConverter148/1 -> bus_creator/161  "VHAL_RrMotorAvailTq_Nm"
  [VHAL_RrMotorAvailTq_Nm] -> UnitConverter148/1
  MCU_R1/24(VHAL_RrRegenAvailTq_Nm) -> [VHAL_RrRegenAvailTq_Nm]
  UnitConverter149/1 -> bus_creator/162  "VHAL_RrRegenAvailTq_Nm"
  [VHAL_RrRegenAvailTq_Nm] -> UnitConverter149/1
  MCU_R1/25(VHAL_RrTMSpd_rpm) -> [VHAL_RrTMSpd_rpm]
  UnitConverter150/1 -> bus_creator/163  "VHAL_RrTMSpd_rpm"
  [VHAL_RrTMSpd_rpm] -> UnitConverter150/1
  MCU_R1/26(VHAL_RrTMTemp_C) -> [VHAL_RrTMTemp_C]
  UnitConverter151/1 -> bus_creator/164  "VHAL_RrTMTemp_C"
  [VHAL_RrTMTemp_C] -> UnitConverter151/1
  MCU_R1/27(VHAL_RrTMid_A) -> [VHAL_RrTMid_A]
  UnitConverter152/1 -> bus_creator/165  "VHAL_RrTMid_A"
  [VHAL_RrTMid_A] -> UnitConverter152/1
  MCU_R1/28(VHAL_RrTMiq_A) -> [VHAL_RrTMiq_A]
  UnitConverter153/1 -> bus_creator/166  "VHAL_RrTMiq_A"
  [VHAL_RrTMiq_A] -> UnitConverter153/1
  VHAL_CANMsgInvalidMCUR2_flg/1(Out) -> bus_creator/167
  MCU_R2/1(VHAL_RrCoolanttempReq_cnt) -> [VHAL_RrCoolanttempReq_cnt]
  UnitConverter154/1 -> bus_creator/168  "VHAL_RrCoolanttempReq_cnt"
  [VHAL_RrCoolanttempReq_cnt] -> UnitConverter154/1
  MCU_R2/2(VHAL_RrEOPSpdSet_rpm) -> [VHAL_RrEOPSpdSet_rpm]
  UnitConverter155/1 -> bus_creator/169  "VHAL_RrEOPSpdSet_rpm"
  [VHAL_RrEOPSpdSet_rpm] -> UnitConverter155/1
  MCU_R2/3(VHAL_RrFailcode1_enum) -> [VHAL_RrFailcode1_enum]
  UnitConverter156/1 -> bus_creator/170  "VHAL_RrFailcode1_enum"
  [VHAL_RrFailcode1_enum] -> UnitConverter156/1
  MCU_R2/4(VHAL_RrFailcode2_enum) -> [VHAL_RrFailcode2_enum]
  UnitConverter157/1 -> bus_creator/171  "VHAL_RrFailcode2_enum"
  [VHAL_RrFailcode2_enum] -> UnitConverter157/1
  MCU_R2/5(VHAL_RrFailcodehistory1_enum) -> [VHAL_RrFailcodehistory1_enum]
  UnitConverter158/1 -> bus_creator/172  "VHAL_RrFailcodehistory1_enum"
  [VHAL_RrFailcodehistory1_enum] -> UnitConverter158/1
  MCU_R2/6(VHAL_RrFailcodehistory2_enum) -> [VHAL_RrFailcodehistory2_enum]
  UnitConverter159/1 -> bus_creator/173  "VHAL_RrFailcodehistory2_enum"
  [VHAL_RrFailcodehistory2_enum] -> UnitConverter159/1
  MCU_R2/7(VHAL_RrLLCTemp_C) -> [VHAL_RrLLCTemp_C]
  UnitConverter160/1 -> bus_creator/174  "VHAL_RrLLCTemp_C"
  [VHAL_RrLLCTemp_C] -> UnitConverter160/1
  MCU_R2/8(VHAL_RrLLCflowReq_Lpmin) -> [VHAL_RrLLCflowReq_Lpmin]
  UnitConverter161/1 -> bus_creator/175  "VHAL_RrLLCflowReq_Lpmin"
  [VHAL_RrLLCflowReq_Lpmin] -> UnitConverter161/1
  MCU_R2/9(VHAL_RrMCUTempWarn_enum) -> [VHAL_RrMCUTempWarn_enum]
  UnitConverter162/1 -> bus_creator/176  "VHAL_RrMCUTempWarn_enum"
  [VHAL_RrMCUTempWarn_enum] -> UnitConverter162/1
  MCU_R2/10(VHAL_RrTMTempWarn_enum) -> [VHAL_RrTMTempWarn_enum]
  UnitConverter163/1 -> bus_creator/177  "VHAL_RrTMTempWarn_enum"
  [VHAL_RrTMTempWarn_enum] -> UnitConverter163/1
  VHAL_CANMsgInvalidShifter1_flg/1(Out) -> bus_creator/178
  Shifter1/1(VHAL_Shifter1CSErr_flg) -> [VHAL_Shifter1CSErr_flg]
  UnitConverter164/1 -> bus_creator/179  "VHAL_Shifter1CSErr_flg"
  [VHAL_Shifter1CSErr_flg] -> UnitConverter164/1
  Shifter1/2(VHAL_Shifter1RCErr_flg) -> [VHAL_Shifter1RCErr_flg]
  UnitConverter165/1 -> bus_creator/180  "VHAL_Shifter1RCErr_flg"
  [VHAL_Shifter1RCErr_flg] -> UnitConverter165/1
  Shifter1/3(VHAL_ShifterCRC8_enum) -> [VHAL_ShifterCRC8_enum]
  UnitConverter166/1 -> bus_creator/181  "VHAL_ShifterCRC8_enum"
  [VHAL_ShifterCRC8_enum] -> UnitConverter166/1
  Shifter1/4(VHAL_ShifterHandleCmd_enum) -> [VHAL_ShifterHandleCmd_enum]
  UnitConverter167/1 -> bus_creator/182  "VHAL_ShifterHandleCmd_enum"
  [VHAL_ShifterHandleCmd_enum] -> UnitConverter167/1
  Shifter1/5(VHAL_ShifterRC_enum) -> [VHAL_ShifterRC_enum]
  UnitConverter168/1 -> bus_creator/183  "VHAL_ShifterRC_enum"
  [VHAL_ShifterRC_enum] -> UnitConverter168/1
